simulink model "FM_RXTX_Test_Sinus_Sound"  (R2020b)
settings: Solver=VariableStepAuto  StartTime=0.0  StopTime=5  RelTol=1e-3
undefined symbols (not defined in the file or in its folder): designMultirateFIR
libraries: commanabbnd3 x2, dspmlti4 x1, dspsrcs4 x1, dspobslib x1
settings Model: Creator=Guillaume  LastModifiedBy=Guillaume

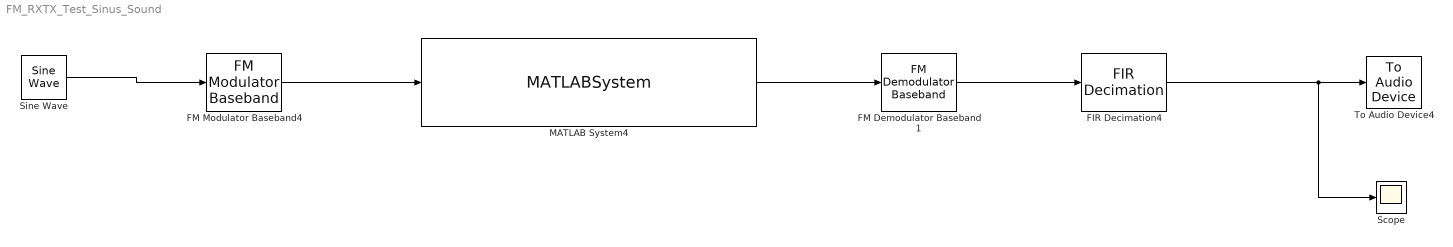
== system FM_RXTX_Test_Sinus_Sound ==
  FIR Decimation4 : dspmlti4/FIR Decimation  FilterSource=Auto  h=designMultirateFIR(1,2)  D=30  filtStruct=Direct form  FilterObject=FDECIM  InputProcessing=Columns as channels (frame based)  framing=Enforce single-rate processing  inputOffset=0  outputBufInitCond=0  roundingMode=Floor  overflowMode=off  firstCoeffDataTypeStr=Inherit: Same word length as input  firstCoeffMin=[]  firstCoeffMax=[]  firstCoeffLastDataTypeStr=Inherit: Same word length as input  outputDataTypeStr=Inherit: Same as accumulator  outputMin=[]  outputMax=[]  outputLastDataTypeStr=Inherit: Same as accumulator
  FM Demodulator Baseband 1 : commanabbnd3/FM Demodulator Baseband   FrequencyDeviation=75e3  SimulateUsing=Code generation
      settings: SourceProductBaseCode=CM
  FM Modulator Baseband4 : commanabbnd3/FM Modulator Baseband  FrequencyDeviation=75e3  SimulateUsing=Code generation
      settings: SourceProductBaseCode=CM
  MATLAB System4 : MATLABSystem  System=limeSDR_Simulink_Wrapper_2022  enable_rx0=on  rx0_antenna=3  rx0_bandwidth=1.5  rx0_gain=10  rx_frequency=868e6  rx_samplerate=1.44e6  rx_timeout_ms=5000  rx_step_size=18000  enable_tx0=on  tx0_antenna=2  tx0_bandwidth=1.5  tx0_gain=10  tx_frequency=868e6  tx_samplerate=1.44e6  tx_timeout_ms=5000  tx_step_size=18000
      mask Type: limeSDR_Simulink_Wrapper_2022
      mask Display:
      | disp('LimeSDR mini');
      | port_label('input',1,'TX0 Samples');
      | port_label('output',1,'RX0 Samples');
  Scope : Scope
  Sine Wave : dspsrcs4/Sine Wave  Amplitude=1  Frequency=440  Phase=0  SampleMode=Discrete  OutComplex=Real  CompMethod=Trigonometric fcn  TableSize=Speed  SampleTime=1/1.44e6  SamplesPerFrame=18000  ResetState=Restart at time zero  OutputFrames=off  dataType=double  wordLen=16  udDataType=sfix(16)  fracBitsMode=Best precision  numFracBits=15  OutDataTypeStr=double  LastOutDataTypeStr=double
  To Audio Device4 : dspobslib/To Audio Device  deviceName=Default  inheritSampleRate=on  sampleRate=44100  deviceDatatype=Determine from input data type  autoBufferSize=on  bufferSize=4096  queueDuration=1.0  defaultOutputChannelMapping=on  outputChannelMapping=1  outputNumUnderrunSamples=off
      settings: SourceProductBaseCode=DS
  wires:
  FM Modulator Baseband4/1 -> MATLAB System4/1
  MATLAB System4/1 -> FM Demodulator Baseband 1/1
  FM Demodulator Baseband 1/1 -> FIR Decimation4/1
  FIR Decimation4/1 -> Scope/1, To Audio Device4/1
  Sine Wave/1 -> FM Modulator Baseband4/1
